simulink model "Longitudinal"  (R2016b)
settings: Solver=VariableStepAuto  StartTime=0.0  StopTime=3000.0  RelTol=1e-3
values from neighbouring files (symbols this model uses):
  Af = 2.8    [Longitudinal_script.m]
  Cd = 0.29    [Longitudinal_script.m]
  Crr = 0.015    [Longitudinal_script.m]
  eff = 0.9    [Longitudinal_script.m]
  g = 9.81    [Longitudinal_script.m]
  Iw = 1    [Longitudinal_script.m]
  lamda = 4.1    [Longitudinal_script.m]
  M = 2458.924    [Longitudinal_script.m]
  Meq = 0.1*M    (= 245.8924)    [Longitudinal_script.m]
  Pa = 1.225    [Longitudinal_script.m]
  Rw = 0.3    [Longitudinal_script.m]
settings Model: Creator=wu.2828  LastModifiedBy=wu.2828

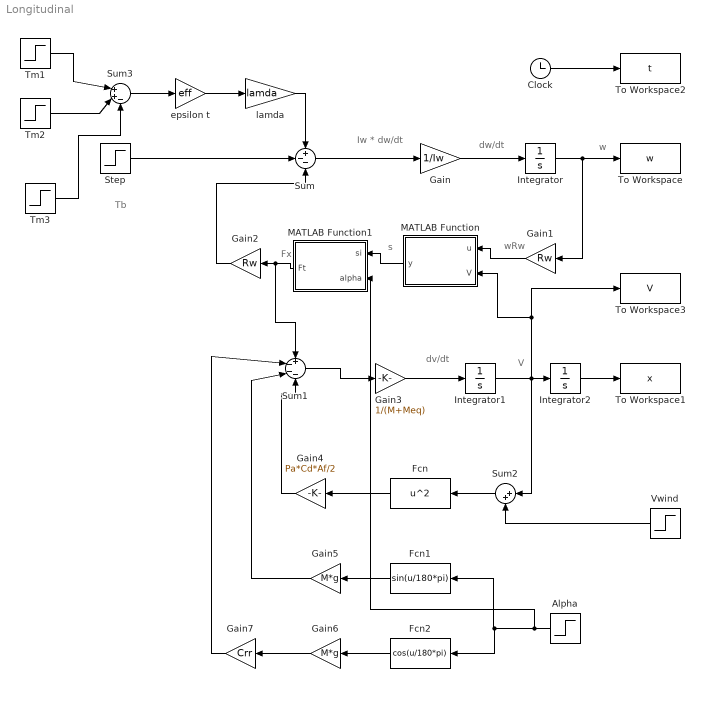
== system Longitudinal ==
  note: Tb
  note: V
  note: dv/dt
  note: Fx
  note: s
  note: wRw
  note: w
  note: dw/dt
  note: Iw * dw/dt
  Alpha : Step  Time=1700  After=0  SampleTime=0
  Clock : Clock
  Fcn : Fcn  Expr=u^2
  Fcn1 : Fcn  Expr=sin(u/180*pi)
  Fcn2 : Fcn  Expr=cos(u/180*pi)
  Gain : Gain  Gain=1/Iw
  Gain1 : Gain  Gain=Rw
  Gain2 : Gain  Gain=Rw
  Gain3 : Gain  Gain=1/(M+Meq)
  Gain4 : Gain  Gain=Pa*Cd*Af/2
  Gain5 : Gain  Gain=M*g
  Gain6 : Gain  Gain=M*g
  Gain7 : Gain  Gain=Crr
  Integrator : Integrator  InitialCondition=0.01
  Integrator1 : Integrator  InitialCondition=0.01
  Integrator2 : Integrator
  MATLAB Function : MATLAB Function  TreatAsAtomicUnit=on
  MATLAB Function1 : MATLAB Function  TreatAsAtomicUnit=on
  Step : Step  Time=1700  After=0  SampleTime=0
  Sum : Sum  Inputs=+--
  Sum1 : Sum  Inputs=+---
  Sum2 : Sum  Inputs=|++
  Sum3 : Sum  Inputs=|++-
  Tm1 : Step  Time=0  After=29  SampleTime=0
  Tm2 : Step  Time=1700  After=0  SampleTime=0
  Tm3 : Step  Time=1700  After=0  SampleTime=0
  To Workspace : ToWorkspace  VariableName=w  SaveFormat=Timeseries  SampleTime=-1
  To Workspace1 : ToWorkspace  VariableName=x  SaveFormat=Timeseries  SampleTime=-1
  To Workspace2 : ToWorkspace  VariableName=t  SaveFormat=Timeseries  SampleTime=-1
  To Workspace3 : ToWorkspace  VariableName=V  SaveFormat=Timeseries  SampleTime=-1
  Vwind : Step  Time=1700  After=10  SampleTime=0
  epsilon t : Gain  Gain=eff
  "lamda " : Gain  Gain=lamda
  wires:
  epsilon t/1 -> "lamda "/1
  "lamda "/1 -> Sum/1
  Sum/1 -> Gain/1
  Gain/1 -> Integrator/1
  Integrator/1 -> To Workspace/1, Gain1/1
  Gain1/1 -> MATLAB Function/1(u)
  MATLAB Function/1(y) -> MATLAB Function1/1(si)
  MATLAB Function1/1(Ft) -> Sum1/1, Gain2/1
  Gain2/1 -> Sum/3
  Sum1/1 -> Gain3/1
  Gain3/1 -> Integrator1/1
  Integrator1/1 -> Sum2/1, To Workspace3/1, MATLAB Function/2(V), Integrator2/1
  Integrator2/1 -> To Workspace1/1
  Vwind/1 -> Sum2/2
  Sum2/1 -> Fcn/1
  Fcn/1 -> Gain4/1
  Gain4/1 -> Sum1/4
  Alpha/1 -> MATLAB Function1/2(alpha), Fcn2/1, Fcn1/1
  Fcn1/1 -> Gain5/1
  Fcn2/1 -> Gain6/1
  Gain5/1 -> Sum1/3
  Gain6/1 -> Gain7/1
  Gain7/1 -> Sum1/2
  Clock/1 -> To Workspace2/1
  Tm1/1 -> Sum3/1
  Tm2/1 -> Sum3/2
  Sum3/1 -> epsilon t/1
  Step/1 -> Sum/2
  Tm3/1 -> Sum3/3

== matlab function Longitudinal/MATLAB Function1 ==
  data: si input; Ft output; alpha input
function Ft = fcn(si,alpha)
m = 2458.924;
g = 9.81 ;
mu = 0.7;    %Dry road friction coeff
Fz = m*g/4; 
C_s = 3e5;
C_alpha = 1.5e5;




    S= mu*Fz*(1-si)./(2*sqrt(C_s^2*si.^2 + C_alpha^2*tand(alpha)^2));             ;%since er=0
    
    if S <1
            f = S.*(2-S);
    else 
            f = 1 ;
    end
    
    Ft = C_s*si.*f./(1-si);

== matlab function Longitudinal/MATLAB Function ==
  data: u input; y output; V input
function y = fcn(u,V)
A = max([V,u]);
y=(u-V)/A;
